simulink subsystem "VehicleLocalPosition"  (R2024a)
settings: Solver=VariableStepAuto  StartTime=0.0  StopTime=10.0  RelTol=1e-3
libraries: uavmavlinklib x1
settings Model: Creator=gurt1  LastModifiedBy=gurt1

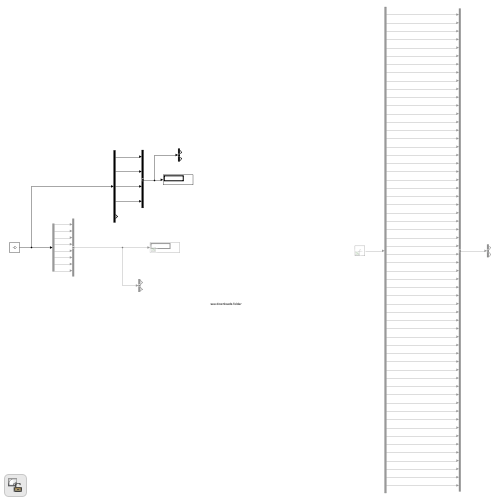
[thumbnail: Simulink's stored preview of the top-level diagram]
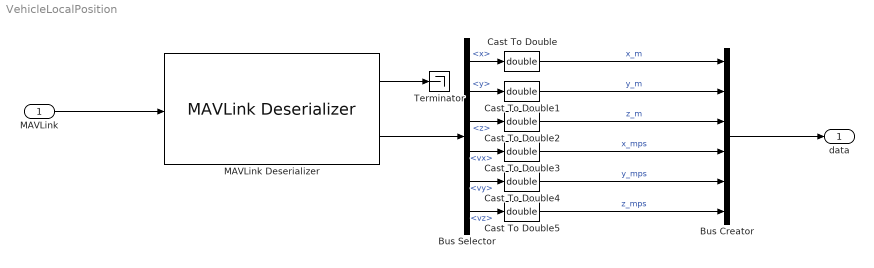
== system VehicleLocalPosition ==
  MAVLink : Inport
  Bus Creator : BusCreator  Inputs=6
  Bus Selector : BusSelector  OutputSignals=Payload.x,Payload.y,Payload.z,Payload.vx,Payload.vy,Payload.vz
  Cast To Double{,1..5} (6 alike) : DataTypeConversion  OutDataTypeStr=double  SaturateOnIntegerOverflow=off  RndMeth=Floor
  MAVLink Deserializer : uavmavlinklib/MAVLink Deserializer  dialectSource=Select from standard MAVLink dialects  dialect=common.xml  dialectCustom=common.xml  version=2  messageType=LOCAL_POSITION_NED  inputDataLength=off  SystemIDFilter=off  systemID=1  ComponentIDFilter=off  componentID=1  queueMsg=off  queueMsgSize=50  dropNum=off
  Terminator : Terminator
  data : Outport
  wires:
  Bus Creator/1 -> data/1
  MAVLink/1 -> MAVLink Deserializer/1
  MAVLink Deserializer/1 -> Terminator/1
  MAVLink Deserializer/2 -> Bus Selector/1
  Bus Selector/1 -> Cast To Double/1  "<x>"
  Bus Selector/2 -> Cast To Double1/1  "<y>"
  Bus Selector/3 -> Cast To Double2/1  "<z>"
  Bus Selector/4 -> Cast To Double3/1  "<vx>"
  Bus Selector/5 -> Cast To Double4/1  "<vy>"
  Bus Selector/6 -> Cast To Double5/1  "<vz>"
  Cast To Double/1 -> Bus Creator/1  "x_m"
  Cast To Double1/1 -> Bus Creator/2  "y_m"
  Cast To Double2/1 -> Bus Creator/3  "z_m"
  Cast To Double3/1 -> Bus Creator/4  "x_mps"
  Cast To Double4/1 -> Bus Creator/5  "y_mps"
  Cast To Double5/1 -> Bus Creator/6  "z_mps"
